simulink subsystem "Body_Frame_Acceleration"  (R2023b)
settings: Solver=VariableStepAuto  StartTime=0.0  StopTime=10.0  RelTol=1e-3
undefined symbols (not defined in the file): g
libraries: matrix_library x1
settings Model: Creator=Andrew Radulovich  LastModifiedBy=thatf
settings ModelReferenceCC: EnableRefExpFcnMdlSchedulingChecks=on

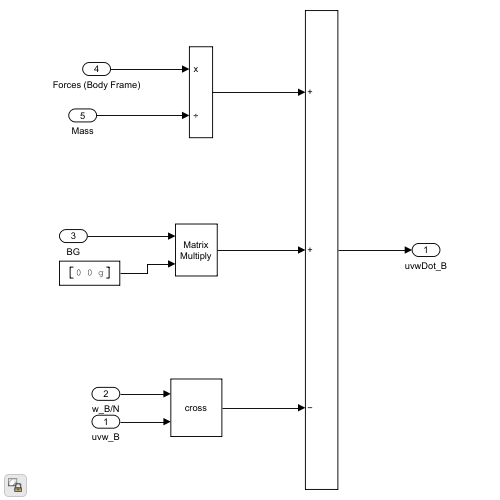
[thumbnail: Simulink's stored preview of the top-level diagram]
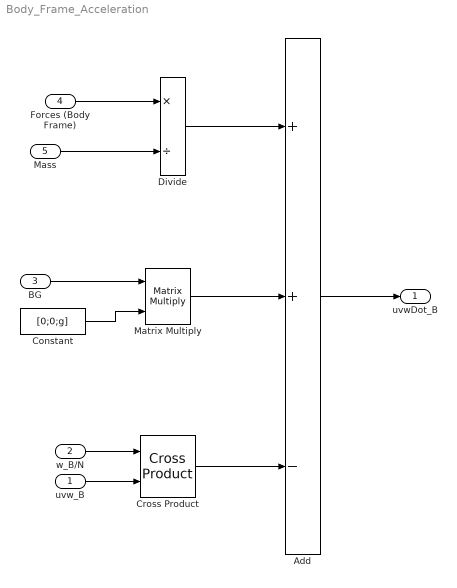
== system Body_Frame_Acceleration ==
  uvw_B : Inport
  w_B/N : Inport  Port=2
  BG : Inport  Port=3
  Forces (Body Frame) : Inport  Port=4
  Mass : Inport  Port=5
  Add : Sum  Inputs=++-
  Constant : Constant  Value=[0;0;g]
  Cross Product : matrix_library/Cross Product
  Divide : Product  Inputs=*/
  Matrix Multiply : Product  Multiplication=Matrix(*)
  uvwDot_B : Outport
  wires:
  Forces (Body Frame)/1 -> Divide/1
  Mass/1 -> Divide/2
  Add/1 -> uvwDot_B/1
  Divide/1 -> Add/1
  w_B/N/1 -> Cross Product/1
  uvw_B/1 -> Cross Product/2
  BG/1 -> Matrix Multiply/1
  Matrix Multiply/1 -> Add/2
  Constant/1 -> Matrix Multiply/2
  Cross Product/1 -> Add/3
